simulink model "LinearAnalysisSM_example"  (R2017a)
settings: Solver=VariableStepAuto  StartTime=0.0  StopTime=20  MaxStep=.1  RelTol=1e-3
undefined symbols (not defined in the file or in its folder): SS
settings Model: Creator=erich  LastModifiedBy=erich

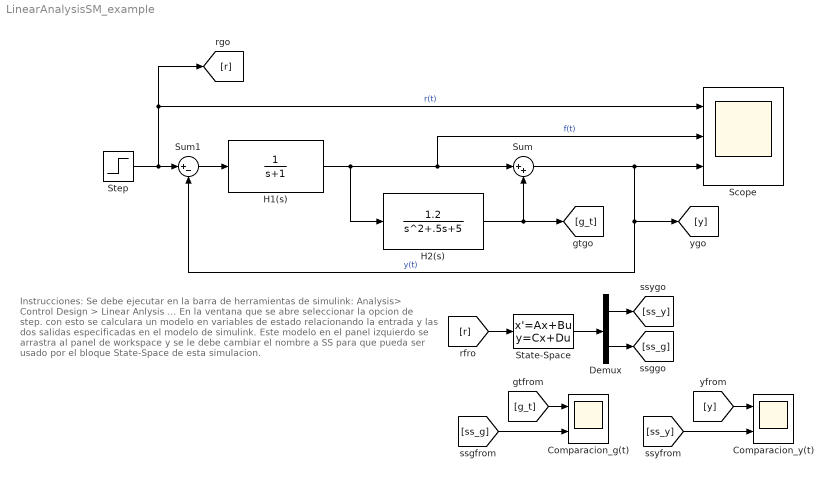
== system LinearAnalysisSM_example ==
  note: Instrucciones:
      | Se debe ejecutar en la barra de herramientas de simulink:
      | Analysis> Control Design > Linear Anlysis ...
      | En la ventana que se abre seleccionar la opcion de step.
      | con esto se calculara un modelo en variables de estado
      | relacionando la entrada y las dos salidas especificadas
      | en el modelo de simulink. Este modelo en el panel izquierdo
      | se arrastra al panel de workspace y se le debe cambiar el
      | nombre a SS para que pueda ser usado por el bloque
      | State-Space de esta simulacion.
  Comparacion_g(t) : Scope  NumInputPorts=2
  Comparacion_y(t) : Scope  NumInputPorts=2
  Demux : Demux  Outputs=2
  H1(s) : TransferFcn  Denominator=[1 1]
  H2(s) : TransferFcn  Numerator=[1.2]  Denominator=[1 .5 5]
  Scope : Scope  NumInputPorts=3
  State-Space : StateSpace  A=SS.A  B=SS.B  C=SS.C  D=SS.D  X0=0
  Step : Step  SampleTime=0
  Sum : Sum  Inputs=|++
  Sum1 : Sum  Inputs=|+-
  wires:
  H1(s)/1 -> H2(s)/1, Scope/2, Sum/1  "f(t)"
  H2(s)/1 -> [g_t], Sum/2
  Step/1 -> Scope/1, [r], Sum1/1  "r(t)"
  Sum1/1 -> H1(s)/1
  Sum/1 -> Scope/3, Sum1/2, [y]  "y(t)"
  [r] -> State-Space/1
  State-Space/1 -> Demux/1
  [g_t] -> Comparacion_g(t)/1
  [ss_g] -> Comparacion_g(t)/2
  [ss_y] -> Comparacion_y(t)/2
  [y] -> Comparacion_y(t)/1
  Demux/1 -> [ss_y]
  Demux/2 -> [ss_g]
